simulink model "Parallel_Resonant_converter"  (R2024b)
settings: Solver=ode4  StartTime=0.0  StopTime=0.1  FixedStep=1e-7  RelTol=1e-3
libraries: spsSeriesRLCBranchLib x5, spsCurrentMeasurementLib x5, spsVoltageMeasurementLib x5, spsDiodeLib x4, spsIGBTDiodeLib x4, spsDCVoltageSourceLib x1, sps_lib x1
settings Model: Creator=adity  LastModifiedBy=adity

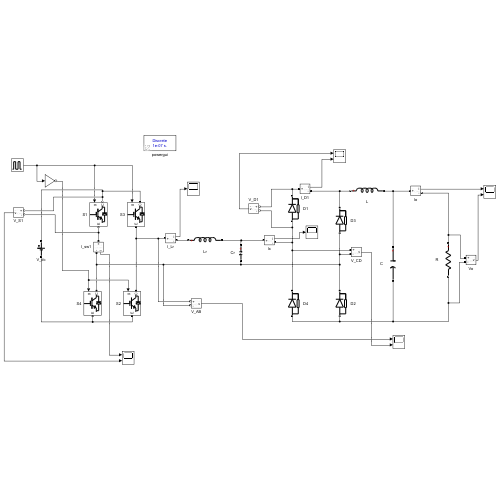
[thumbnail: Simulink's stored preview of the top-level diagram]
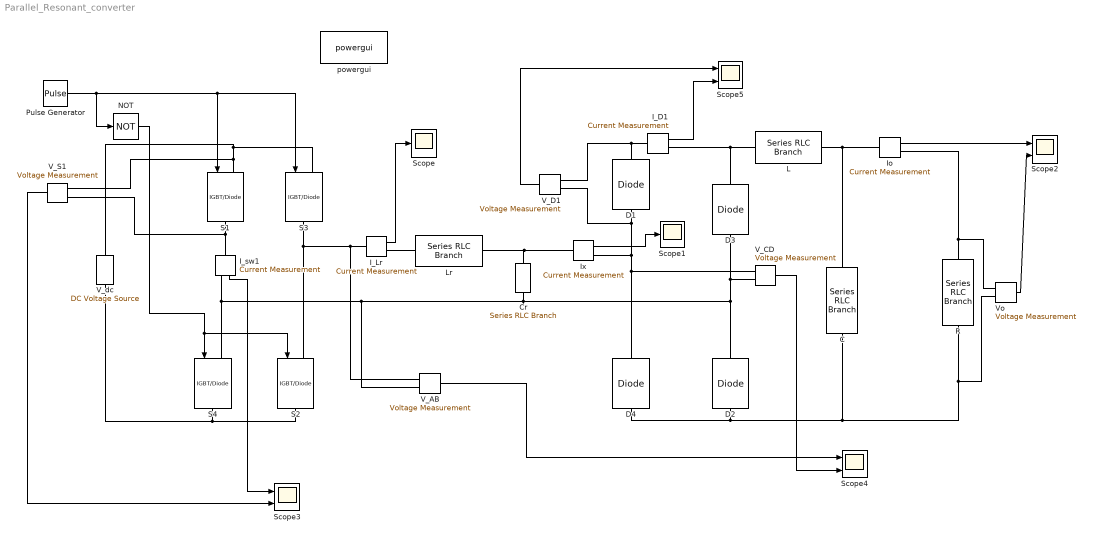
== system Parallel_Resonant_converter ==
  C : spsSeriesRLCBranchLib/Series RLC Branch  LConnTagsString=__new0  RConnTagsString=__new0  BranchType=C  Resistance=1  Inductance=1e-3  SetiL0=off  InitialCurrent=0  Capacitance=2.35e-6  Setx0=off  InitialVoltage=0  Measurements=None
  Cr : spsSeriesRLCBranchLib/Series RLC Branch  LConnTagsString=__new0  RConnTagsString=__new0  BranchType=C  Resistance=1  Inductance=1e-3  SetiL0=off  InitialCurrent=0  Capacitance=24.5e-9  Setx0=off  InitialVoltage=0  Measurements=Branch voltage
  D{1..4} (4 alike) : spsDiodeLib/Diode  Ron=0.000001  Lon=0  Vf=0  IC=0  UseSnubber=0  Rs=500  Cs=250e-9  Measurements=off
  I_D1 : spsCurrentMeasurementLib/Current Measurement  PhasorSimulation=off  OutputType=Complex  PSBequivalent=0
  I_Lr : spsCurrentMeasurementLib/Current Measurement  PhasorSimulation=off  OutputType=Complex  PSBequivalent=0
  I_sw1 : spsCurrentMeasurementLib/Current Measurement  PhasorSimulation=off  OutputType=Complex  PSBequivalent=0
  Io : spsCurrentMeasurementLib/Current Measurement  PhasorSimulation=off  OutputType=Complex  PSBequivalent=0
  Ix : spsCurrentMeasurementLib/Current Measurement  PhasorSimulation=off  OutputType=Complex  PSBequivalent=0
  L : spsSeriesRLCBranchLib/Series RLC Branch  LConnTagsString=__new0  RConnTagsString=__new0  BranchType=L  Resistance=1  Inductance=80e-6  SetiL0=off  InitialCurrent=0  Capacitance=1e-6  Setx0=off  InitialVoltage=0  Measurements=Branch voltage and current
  Lr : spsSeriesRLCBranchLib/Series RLC Branch  LConnTagsString=__new0  RConnTagsString=__new0  BranchType=L  Resistance=1  Inductance=264.6e-6  SetiL0=off  InitialCurrent=0  Capacitance=1e-6  Setx0=off  InitialVoltage=0  Measurements=Branch voltage and current
  NOT : Logic  Operator=NOT  IconShape=distinctive  AllPortsSameDT=off  OutDataTypeStr=boolean
  Pulse Generator : DiscretePulseGenerator  PulseType=Time based  Period=1/(250e3)  PulseWidth=50
  R : spsSeriesRLCBranchLib/Series RLC Branch  LConnTagsString=__new0  RConnTagsString=__new0  BranchType=R  Resistance=1  Inductance=1e-3  SetiL0=off  InitialCurrent=0  Capacitance=1e-6  Setx0=off  InitialVoltage=0  Measurements=Branch voltage and current
  S{1..4} (4 alike) : spsIGBTDiodeLib/IGBT//Diode  Ron=1e-5  Rs=1e5  Cs=inf  Measurements=off
  Scope : Scope
  Scope1 : Scope
  Scope{2..5} (4 alike) : Scope  NumInputPorts=2
  V_AB : spsVoltageMeasurementLib/Voltage Measurement  PhasorSimulation=off  OutputType=Complex  PSBequivalent=0
  V_CD : spsVoltageMeasurementLib/Voltage Measurement  PhasorSimulation=off  OutputType=Complex  PSBequivalent=0
  V_D1 : spsVoltageMeasurementLib/Voltage Measurement  PhasorSimulation=off  OutputType=Complex  PSBequivalent=0
  V_S1 : spsVoltageMeasurementLib/Voltage Measurement  PhasorSimulation=off  OutputType=Complex  PSBequivalent=0
  V_dc : spsDCVoltageSourceLib/DC Voltage Source  Amplitude=12  Measurements=None
  Vo : spsVoltageMeasurementLib/Voltage Measurement  PhasorSimulation=off  OutputType=Complex  PSBequivalent=0
  powergui : sps_lib/powergui  Priority=1  SimulationMode=Discrete  SampleTime=1e-7  frequency=60  Iterations=50  frequencyindice=0  Pbase=100e6  ErrMax=1e-4  UnitsV=kV  UnitsW=MW  buscounter=0  FunctionMessages=off  echomessages=off  EnableUseOfTLC=off  CurrentSourceSwitches=off  DisableSnubberDevices=off  DisableRonSwitches=off  DisableVfSwitches=off  DisplayEquations=off  AutomaticDiscreteSolvers=off  SolverType=Tustin/Backward Euler (TBE)  Interpol=off  ExternalGateDelay=off  methode=off  Ts=100  x0status=blocks  SPID=on  SwTol=0  HookPort=off  NonlinearTolerance=1e-4  nMaxIteration=100  ContinueOnMaxIteration=off  RestoreLinks=warning  ResistiveCurrentMeasurement=off  Frange=[0:2:500]  Ylog=off  Xlog=on  ShowGrid=off  save=off  variable=ZData  structure=0  ZoomFFT=off  StartTime=0.0  cycles=1  DisplayStyle=1  fundamental=60  FreqAxis=off  MaxFrequency=1000  frequencyindicesteady=1  RmsSteady=1  display=off
  wires:
  V_CD/1 -> Scope4/2
  Vo/1 -> Scope2/2
  V_AB/1 -> Scope4/1
  Pulse Generator/1 -> S3/1, S1/1, NOT/1
  I_Lr/1 -> Scope/1
  Io/1 -> Scope2/1
  I_sw1/1 -> Scope3/1
  V_S1/1 -> Scope3/2
  I_D1/1 -> Scope5/2
  V_D1/1 -> Scope5/1
  Ix/1 -> Scope1/1
  NOT/1 -> S2/1, S4/1
  connections:
  I_D1/LConn1 -- D1/RConn1 -- V_D1/LConn1
  Io/LConn1 -- L/RConn1 -- C/LConn1
  V_CD/LConn1 -- D4/RConn1 -- Ix/RConn1 -- V_D1/LConn2 -- D1/LConn1
  D2/RConn1 -- Cr/RConn1 -- S4/LConn1 -- I_sw1/RConn1 -- V_AB/LConn2 -- D3/LConn1 -- V_CD/LConn2
  R/RConn1 -- Vo/LConn2 -- C/RConn1 -- D4/LConn1 -- D2/LConn1
  Lr/LConn1 -- I_Lr/RConn1
  R/LConn1 -- Io/RConn1 -- Vo/LConn1
  S3/RConn1 -- I_Lr/LConn1 -- V_AB/LConn1 -- S2/LConn1
  V_S1/LConn1 -- S3/LConn1 -- V_dc/RConn1 -- S1/LConn1
  Cr/LConn1 -- Ix/LConn1 -- Lr/RConn1
  S4/RConn1 -- S2/RConn1 -- V_dc/LConn1
  S1/RConn1 -- I_sw1/LConn1 -- V_S1/LConn2
  I_D1/RConn1 -- L/LConn1 -- D3/RConn1
